simulink model "pid_zichuang"  (R2021b)
settings: Solver=VariableStepAuto  StartTime=0.0  StopTime=20  RelTol=1e-3
settings Model: Creator=84232  LastModifiedBy=84232
settings SolverCC: ShapePreserveControl=EnableAll

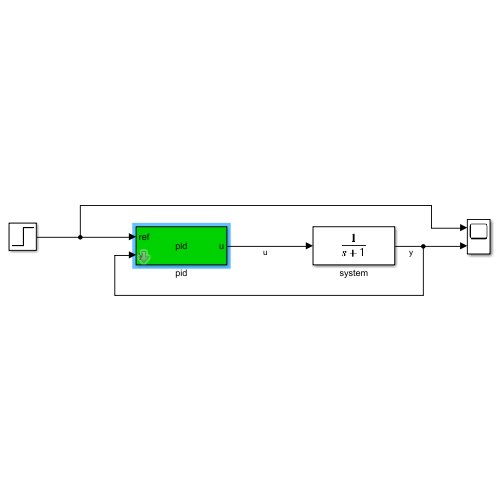
[thumbnail: Simulink's stored preview of the top-level diagram]
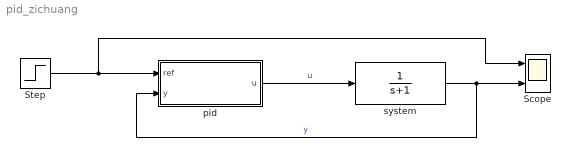
== system pid_zichuang ==
  Scope : Scope  NumInputPorts=2
  Step : Step  SampleTime=0
  pid : Subsystem  mask{kp=1, kd=1, ki=1}
      mask prompts: kp "value-kp"; kd "value-kd"; ki "value-ki"
      mask help: pid controller
      mask Display:
      | disp('pid')
      | port_label('input',1,'ref');
      | port_label('input',2,'y');
      | port_label('output',1,'u');
  system : TransferFcn  Denominator=[1 1]
  wires:
  system/1 -> Scope/2, pid/2(y)  "y"
  pid/1(u) -> system/1  "u"
  Step/1 -> Scope/1, pid/1(ref)

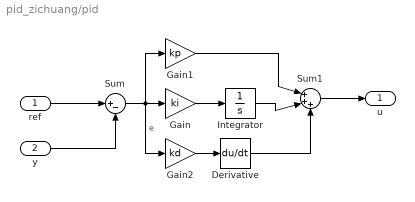
== system pid_zichuang/pid ==
  ref : Inport
  y : Inport  Port=2
  Derivative : Derivative
  Gain : Gain  Gain=ki
  Gain1 : Gain  Gain=kp
  Gain2 : Gain  Gain=kd
  Integrator : Integrator
  Sum : Sum  Inputs=|+-
  Sum1 : Sum  Inputs=|+++
  u : Outport
  wires:
  ref/1 -> Sum/1
  y/1 -> Sum/2
  Gain/1 -> Integrator/1
  Integrator/1 -> Sum1/2
  Sum/1 -> Gain2/1, Gain1/1, Gain/1  "e"
  Gain2/1 -> Derivative/1
  Derivative/1 -> Sum1/3
  Gain1/1 -> Sum1/1
  Sum1/1 -> u/1
